simulink model "bh_explore_speed_control_and_manoeuvres"  (R2018a)
settings: Solver=ode45  StartTime=0.0  StopTime=15  FixedStep=0.001  RelTol=1e-5
undefined symbols (not defined in the file or in its folder): sigbuilder_block
libraries: simulink_extras x14, bh_cv_car_drc_library x1
settings Model: Creator=bhorton  LastModifiedBy=bhorton
settings SolverCC: ZeroCrossControl=EnableAll  ZeroCrossAlgorithm=Adaptive
settings DebuggingCC: SignalInfNanChecking=warning
settings ModelReferenceCC: ModelReferenceMinAlgLoopOccurrences=on

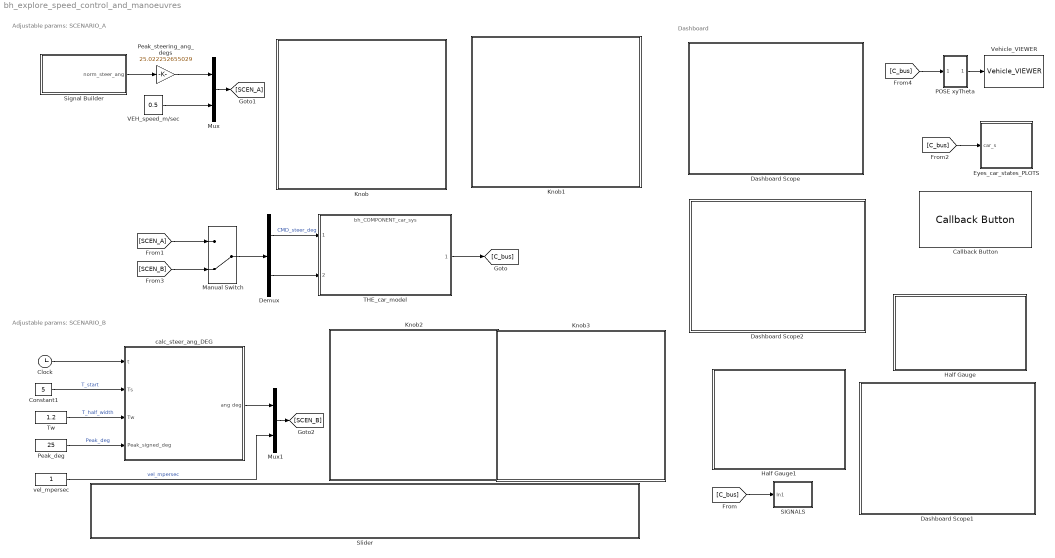
== system bh_explore_speed_control_and_manoeuvres ==
  note: Dashboard
  note: Adjustable params: SCENARIO_A
  note: Adjustable params: SCENARIO_B
  Callback Button : CallbackButton  WebBlockId=1673  PressFcn=""  ButtonText=OPEN State Plots
      settings: ClickFcn=|
      | open_system([bdroot,'/Eyes_car_states_PLOTS/car_states'])
      | open_system([bdroot,'/Eyes_car_states_PLOTS/Forces_BODY_frame'])
  Clock : Clock
  Constant1 : Constant  Value=5
  Dashboard Scope : Subsystem  DialogController=hmiCreateDDGDialog  IsWebBlock=on  mask(MWDashboardBlock){webBlockId=37415055-6488-43ff-9aef-d1c13ce01a1d, webBlockType=sdiscope, ShowInitialText=on, HMISrcModelName=bh_explore_speed_control_and_manoeuvres}
      mask prompts: webBlockId "WebBlock Id"; webBlockType "WebBlock Type"; HMISrcModelName "Source Model"
      mask help: SimulinkHMI:dialogs:HMIScopeDialogDesc
      mask Help: helpview([docroot '/mapfiles/simulink.map'], 'hmi_scope')
      mask Display:
      | if strcmp(get_param(bdroot(gcb),'BlockDiagramType'), 'library')
      |     image([(matlabroot) '/toolbox/simulink/hmi/icons/DashboardScope.png']);
      | end
  Dashboard Scope1 : Subsystem  DialogController=hmiCreateDDGDialog  IsWebBlock=on  mask(MWDashboardBlock){webBlockId=0f87227d-f9f9-4bc4-b6ae-007699aa5c2c, webBlockType=sdiscope, ShowInitialText=on, HMISrcModelName=bh_explore_speed_control_and_manoeuvres}
      mask prompts: webBlockId "WebBlock Id"; webBlockType "WebBlock Type"; HMISrcModelName "Source Model"
      mask help: SimulinkHMI:dialogs:HMIScopeDialogDesc
      mask Help: helpview([docroot '/mapfiles/simulink.map'], 'hmi_scope')
      mask Display:
      | if strcmp(get_param(bdroot(gcb),'BlockDiagramType'), 'library')
      |     image([(matlabroot) '/toolbox/simulink/hmi/icons/DashboardScope.png']);
      | end
  Dashboard Scope2 : Subsystem  DialogController=hmiCreateDDGDialog  IsWebBlock=on  mask(MWDashboardBlock){webBlockId=6b014668-cd52-46a0-a1ab-7f5af930874b, webBlockType=sdiscope, ShowInitialText=on, HMISrcModelName=bh_explore_speed_control_and_manoeuvres}
      mask prompts: webBlockId "WebBlock Id"; webBlockType "WebBlock Type"; HMISrcModelName "Source Model"
      mask help: SimulinkHMI:dialogs:HMIScopeDialogDesc
      mask Help: helpview([docroot '/mapfiles/simulink.map'], 'hmi_scope')
      mask Display:
      | if strcmp(get_param(bdroot(gcb),'BlockDiagramType'), 'library')
      |     image([(matlabroot) '/toolbox/simulink/hmi/icons/DashboardScope.png']);
      | end
  Demux : Demux  Outputs=2
  Eyes_car_states_PLOTS : Subsystem
  Half Gauge : Subsystem  DialogController=hmiCreateDDGDialog  IsWebBlock=on  mask(MWDashboardBlock){webBlockId=7d5ce28d-d875-432d-8f3a-719b52f1dd3d, webBlockType=semicirculargauge, ShowInLibBrowser=on, ShowInitialText=on, HMISrcModelName=bh_explore_speed_control_and_manoeuvres}
      mask prompts: webBlockId "WebBlock Id"; webBlockType "WebBlock Type"; HMISrcModelName "Source Model"
      mask help: SimulinkHMI:dialogs:SemicircularGaugeDialogDesc
      mask Help: helpview([docroot '/mapfiles/simulink.map'], 'hmi_half_gauge')
      mask Display:
      | if strcmp(get_param(bdroot(gcb),'BlockDiagramType'), 'library')
      |     image([(matlabroot) '/toolbox/simulink/hmi/icons/SemicircularGauge.png']);
      | end
  Half Gauge1 : Subsystem  DialogController=hmiCreateDDGDialog  IsWebBlock=on  mask(MWDashboardBlock){webBlockId=b5d4b91a-5326-4bfa-bfd5-f4d409ef95d8, webBlockType=semicirculargauge, ShowInLibBrowser=on, ShowInitialText=on, HMISrcModelName=bh_explore_speed_control_and_manoeuvres}
      mask prompts: webBlockId "WebBlock Id"; webBlockType "WebBlock Type"; HMISrcModelName "Source Model"
      mask help: SimulinkHMI:dialogs:SemicircularGaugeDialogDesc
      mask Help: helpview([docroot '/mapfiles/simulink.map'], 'hmi_half_gauge')
      mask Display:
      | if strcmp(get_param(bdroot(gcb),'BlockDiagramType'), 'library')
      |     image([(matlabroot) '/toolbox/simulink/hmi/icons/SemicircularGauge.png']);
      | end
  Knob : Subsystem  DialogController=hmiCreateDDGDialog  IsWebBlock=on  mask(MWDashboardBlock){webBlockId=3ae3ec89-5f06-4569-b08b-ae0e4db549b5, webBlockType=continuousknob, ShowInLibBrowser=on, ShowInitialText=on, HMISrcModelName=bh_explore_speed_control_and_manoeuvres}
      mask prompts: webBlockId "WebBlock Id"; webBlockType "WebBlock Type"; HMISrcModelName "Source Model"
      mask help: SimulinkHMI:dialogs:ContinuousKnobDialogDesc
      mask Help: helpview([docroot '/mapfiles/simulink.map'], 'hmi_knob')
      mask Display:
      | if strcmp(get_param(bdroot(gcb),'BlockDiagramType'), 'library')
      |     image([(matlabroot) '/toolbox/simulink/hmi/icons/ContinuousKnob.png']);
      | end
  Knob1 : Subsystem  DialogController=hmiCreateDDGDialog  IsWebBlock=on  mask(MWDashboardBlock){webBlockId=ad926c90-b8a8-45cf-ba7e-52fdfa91ce01, webBlockType=continuousknob, ShowInLibBrowser=on, ShowInitialText=on, HMISrcModelName=bh_explore_speed_control_and_manoeuvres}
      mask prompts: webBlockId "WebBlock Id"; webBlockType "WebBlock Type"; HMISrcModelName "Source Model"
      mask help: SimulinkHMI:dialogs:ContinuousKnobDialogDesc
      mask Help: helpview([docroot '/mapfiles/simulink.map'], 'hmi_knob')
      mask Display:
      | if strcmp(get_param(bdroot(gcb),'BlockDiagramType'), 'library')
      |     image([(matlabroot) '/toolbox/simulink/hmi/icons/ContinuousKnob.png']);
      | end
  Knob2 : Subsystem  DialogController=hmiCreateDDGDialog  IsWebBlock=on  mask(MWDashboardBlock){webBlockId=2668dcc9-a1cd-4bf1-9da4-0c933115db1b, webBlockType=continuousknob, ShowInLibBrowser=on, ShowInitialText=on, HMISrcModelName=bh_explore_speed_control_and_manoeuvres}
      mask prompts: webBlockId "WebBlock Id"; webBlockType "WebBlock Type"; HMISrcModelName "Source Model"
      mask help: SimulinkHMI:dialogs:ContinuousKnobDialogDesc
      mask Help: helpview([docroot '/mapfiles/simulink.map'], 'hmi_knob')
      mask Display:
      | if strcmp(get_param(bdroot(gcb),'BlockDiagramType'), 'library')
      |     image([(matlabroot) '/toolbox/simulink/hmi/icons/ContinuousKnob.png']);
      | end
  Knob3 : Subsystem  DialogController=hmiCreateDDGDialog  IsWebBlock=on  mask(MWDashboardBlock){webBlockId=14dcc02d-a3fe-4bd7-90d9-1a858d2b9cd1, webBlockType=continuousknob, ShowInLibBrowser=on, ShowInitialText=on, HMISrcModelName=bh_explore_speed_control_and_manoeuvres}
      mask prompts: webBlockId "WebBlock Id"; webBlockType "WebBlock Type"; HMISrcModelName "Source Model"
      mask help: SimulinkHMI:dialogs:ContinuousKnobDialogDesc
      mask Help: helpview([docroot '/mapfiles/simulink.map'], 'hmi_knob')
      mask Display:
      | if strcmp(get_param(bdroot(gcb),'BlockDiagramType'), 'library')
      |     image([(matlabroot) '/toolbox/simulink/hmi/icons/ContinuousKnob.png']);
      | end
  Manual Switch : ManualSwitch  CurrentSetting=0
  Mux : Mux  Inputs=2
  Mux1 : Mux  Inputs=2
  POSE xyTheta : Subsystem
  Peak_deg : Constant  Value=25
  Peak_steering_ang_degs : Gain  Gain=25.022252655029
  SIGNALS : Subsystem
  Signal Builder : Subsystem  Tag=STV Subsys  LoadFcn=sigbuilder_block('load');  StartFcn=sigbuilder_block('start');  StopFcn=sigbuilder_block('stop');  ClipboardFcn=sigbuilder_block('clipboard');  mask(Sigbuilder block){tuvar=[0:10]}
      mask help: Simulink:masks:SigbuilderBlock_MD
      mask init:
      | if ~strcmp(get_param(bdroot(gcbh),'SimulationStatus'),'stopped') tuvar = sigbuilder_block('maskInit'); end
      settings: CopyFcn=sigbuilder_block('copy');  DeleteFcn=sigbuilder_block('delete');  ModelCloseFcn=sigbuilder_block('modelClose');  PreSaveFcn=sigbuilder_block('preSave');  PauseFcn=sigbuilder_block('pause');  ContinueFcn=sigbuilder_block('continue');  NameChangeFcn=sigbuilder_block('namechange');  OpenFcn=sigbuilder_block('open',[6 24.75 1428 637.5 ]);  CloseFcn=sigbuilder_block('close');
      mask Display: plot(0, 0, 100, 100,[2, 2, 32, 32, 2], [68, 8, 8, 68, 68],[32, 2], [38, 38], [32, 19, 2],[53, 60, 44], [32, 17, 17, 2],[16, 16, 31, 31]);txt = getActiveGroup(gcbh);text(2, 100, txt,'verticalAlignment', 'top');
  Slider : Subsystem  DialogController=hmiCreateDDGDialog  IsWebBlock=on  mask(MWDashboardBlock){webBlockId=1f65ddbe-eef6-400e-a434-9b8f03db9885, webBlockType=slider, ShowInLibBrowser=on, ShowInitialText=on, HMISrcModelName=bh_explore_speed_control_and_manoeuvres}
      mask prompts: webBlockId "WebBlock Id"; webBlockType "WebBlock Type"; HMISrcModelName "Source Model"
      mask help: SimulinkHMI:dialogs:SliderDialogDesc
      mask Help: helpview([docroot '/mapfiles/simulink.map'], 'hmi_slider')
      mask Display:
      | if strcmp(get_param(bdroot(gcb),'BlockDiagramType'), 'library')
      |     image([(matlabroot) '/toolbox/simulink/hmi/icons/Slider.png']);
      | end
  THE_car_model : ModelReference  ModelNameDialog=bh_COMPONENT_car_sys  SimulationMode=Normal  ModelReferenceVersion=1.273
  Tw : Constant  Value=1.2
  VEH_speed_m/sec : Constant  Value=0.5
  Vehicle_VIEWER : bh_cv_car_drc_library/CAR_things/Vehicle_VIEWER  wp_mat=[-1, -1; 2,2]  veh_ID_num=1  veh_init_xytheta=[0,0,0]  Ts=0.1
  calc_steer_ang_DEG : Subsystem
      mask Display: image(imread('evassive_PIC_01.JPG'))
  vel_mpersec : Constant
  wires:
  [C_bus] -> Eyes_car_states_PLOTS/1(car_s)
  THE_car_model/1 -> [C_bus]
  [C_bus] -> POSE xyTheta/1(In1)
  POSE xyTheta/1(Out1) -> Vehicle_VIEWER/1
  Signal Builder/1(norm_steer_ang) -> Peak_steering_ang_degs/1
  Peak_steering_ang_degs/1 -> Mux/1
  [C_bus] -> SIGNALS/1(In1)
  VEH_speed_m/sec/1 -> Mux/2
  Manual Switch/1 -> Demux/1
  Demux/1 -> THE_car_model/1  "CMD_steer_deg"
  Demux/2 -> THE_car_model/2
  [SCEN_A] -> Manual Switch/1
  Mux/1 -> [SCEN_A]
  Peak_deg/1 -> calc_steer_ang_DEG/4(Peak_signed_deg)  "Peak_deg"
  Constant1/1 -> calc_steer_ang_DEG/2(Ts)  "T_start"
  Clock/1 -> calc_steer_ang_DEG/1(t)
  Mux1/1 -> [SCEN_B]
  calc_steer_ang_DEG/1(ang deg) -> Mux1/1
  vel_mpersec/1 -> Mux1/2  "vel_mpersec"
  Tw/1 -> calc_steer_ang_DEG/3(Tw)  "T_half_width"
  [SCEN_B] -> Manual Switch/2

== system bh_explore_speed_control_and_manoeuvres/Dashboard Scope ==

== system bh_explore_speed_control_and_manoeuvres/Dashboard Scope1 ==

== system bh_explore_speed_control_and_manoeuvres/Dashboard Scope2 ==

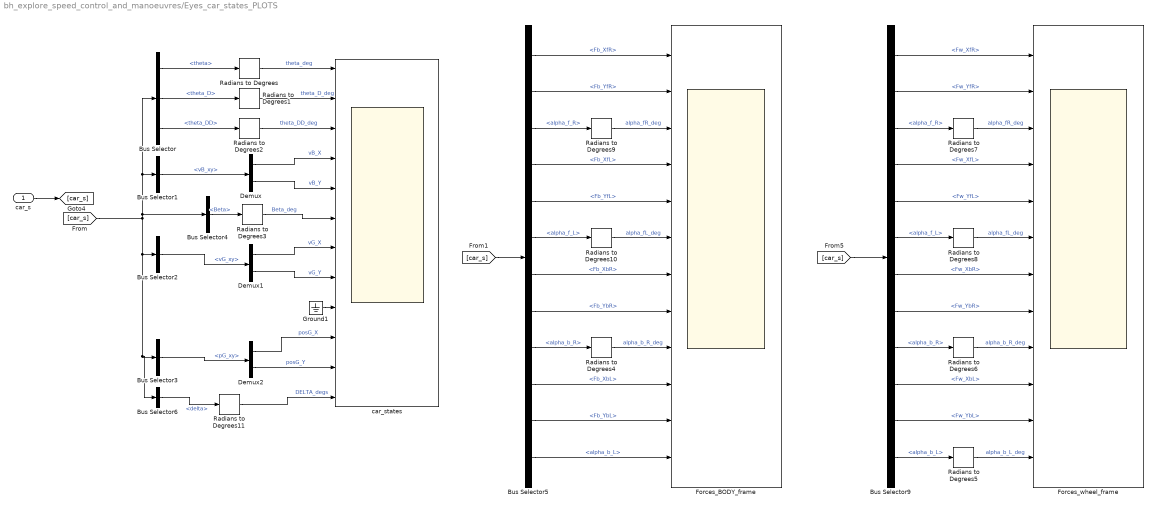
== system bh_explore_speed_control_and_manoeuvres/Eyes_car_states_PLOTS ==
  car_s : Inport
  Bus Selector : BusSelector  OutputSignals=states_B.theta,states_B.theta_D,states_B.theta_DD
  Bus Selector1 : BusSelector  OutputSignals=states_B.vB_xy
  Bus Selector2 : BusSelector  OutputSignals=states_G.vG_xy
  Bus Selector3 : BusSelector  OutputSignals=states_G.pG_xy
  Bus Selector4 : BusSelector  OutputSignals=states_B.Beta
  Bus Selector5 : BusSelector  OutputSignals=Force_BODY_frame.Fb_XfR,Force_BODY_frame.Fb_YfR,alpha.alpha_f_R,Force_BODY_frame.Fb_XfL,Force_BODY_frame.Fb_YfL,alpha.alpha_f_L,Force_BODY_frame.Fb_XbR,Force_BODY_frame.Fb_YbR,alpha.alpha_b_R,Force_BODY_frame.Fb_XbL,Force_BODY_frame.Fb_YbL,alpha.alpha_b_L
  Bus Selector6 : BusSelector  OutputSignals=wheel.delta
  Bus Selector9 : BusSelector  OutputSignals=Force_wheel_frame.Fw_XfR,Force_wheel_frame.Fw_YfR,alpha.alpha_f_R,Force_wheel_frame.Fw_XfL,Force_wheel_frame.Fw_YfL,alpha.alpha_f_L,Force_wheel_frame.Fw_XbR,Force_wheel_frame.Fw_YbR,alpha.alpha_b_R,Force_wheel_frame.Fw_XbL,Force_wheel_frame.Fw_YbL,alpha.alpha_b_L
  Demux : Demux  Outputs=2
  Demux1 : Demux  Outputs=2
  Demux2 : Demux  Outputs=2
  Forces_BODY_frame : Scope  NumInputPorts=12
  Forces_wheel_frame : Scope  NumInputPorts=12
  Ground1 : Ground
  Radians to Degrees{,1..11} (12 alike) : simulink_extras/Transformations/Radians to Degrees
  car_states : Scope  NumInputPorts=12
  wires:
  car_s/1 -> [car_s]
  [car_s] -> Bus Selector4/1, Bus Selector/1, Bus Selector1/1, Bus Selector6/1, Bus Selector3/1, Bus Selector2/1
  Bus Selector/1 -> Radians to Degrees/1  "<theta>"
  Bus Selector/2 -> Radians to Degrees1/1  "<theta_D>"
  Bus Selector/3 -> Radians to Degrees2/1  "<theta_DD>"
  Radians to Degrees/1 -> car_states/1  "theta_deg"
  Radians to Degrees1/1 -> car_states/2  "theta_D_deg"
  Radians to Degrees2/1 -> car_states/3  "theta_DD_deg"
  Bus Selector1/1 -> Demux/1  "<vB_xy>"
  Demux/1 -> car_states/4  "vB_X"
  Demux/2 -> car_states/5  "vB_Y"
  Radians to Degrees3/1 -> car_states/6  "Beta_deg"
  Bus Selector2/1 -> Demux1/1  "<vG_xy>"
  Demux1/1 -> car_states/7  "vG_X"
  Demux1/2 -> car_states/8  "vG_Y"
  Ground1/1 -> car_states/9
  Demux2/1 -> car_states/10  "posG_X"
  Demux2/2 -> car_states/11  "posG_Y"
  Bus Selector3/1 -> Demux2/1  "<pG_xy>"
  Radians to Degrees11/1 -> car_states/12  "DELTA_degs"
  Bus Selector4/1 -> Radians to Degrees3/1  "<Beta>"
  [car_s] -> Bus Selector9/1
  Bus Selector9/1 -> Forces_wheel_frame/1  "<Fw_XfR>"
  Bus Selector9/2 -> Forces_wheel_frame/2  "<Fw_YfR>"
  Bus Selector9/3 -> Radians to Degrees7/1  "<alpha_f_R>"
  Bus Selector9/4 -> Forces_wheel_frame/4  "<Fw_XfL>"
  Bus Selector9/5 -> Forces_wheel_frame/5  "<Fw_YfL>"
  Bus Selector9/6 -> Radians to Degrees8/1  "<alpha_f_L>"
  Bus Selector9/7 -> Forces_wheel_frame/7  "<Fw_XbR>"
  Bus Selector9/8 -> Forces_wheel_frame/8  "<Fw_YbR>"
  Bus Selector9/9 -> Radians to Degrees6/1  "<alpha_b_R>"
  Bus Selector9/10 -> Forces_wheel_frame/10  "<Fw_XbL>"
  Bus Selector9/11 -> Forces_wheel_frame/11  "<Fw_YbL>"
  Bus Selector9/12 -> Radians to Degrees5/1  "<alpha_b_L>"
  Radians to Degrees7/1 -> Forces_wheel_frame/3  "alpha_fR_deg"
  Radians to Degrees8/1 -> Forces_wheel_frame/6  "alpha_fL_deg"
  Radians to Degrees6/1 -> Forces_wheel_frame/9  "alpha_b_R_deg"
  Radians to Degrees5/1 -> Forces_wheel_frame/12  "alpha_b_L_deg"
  Radians to Degrees10/1 -> Forces_BODY_frame/6  "alpha_fL_deg"
  Radians to Degrees4/1 -> Forces_BODY_frame/9  "alpha_b_R_deg"
  Radians to Degrees9/1 -> Forces_BODY_frame/3  "alpha_fR_deg"
  Bus Selector5/9 -> Radians to Degrees4/1  "<alpha_b_R>"
  Bus Selector5/7 -> Forces_BODY_frame/7  "<Fb_XbR>"
  Bus Selector5/10 -> Forces_BODY_frame/10  "<Fb_XbL>"
  Bus Selector5/11 -> Forces_BODY_frame/11  "<Fb_YbL>"
  Bus Selector5/6 -> Radians to Degrees10/1  "<alpha_f_L>"
  Bus Selector5/5 -> Forces_BODY_frame/5  "<Fb_YfL>"
  Bus Selector5/4 -> Forces_BODY_frame/4  "<Fb_XfL>"
  Bus Selector5/8 -> Forces_BODY_frame/8  "<Fb_YbR>"
  Bus Selector5/2 -> Forces_BODY_frame/2  "<Fb_YfR>"
  [car_s] -> Bus Selector5/1
  Bus Selector5/3 -> Radians to Degrees9/1  "<alpha_f_R>"
  Bus Selector5/1 -> Forces_BODY_frame/1  "<Fb_XfR>"
  Bus Selector5/12 -> Forces_BODY_frame/12  "<alpha_b_L>"
  Bus Selector6/1 -> Radians to Degrees11/1  "<delta>"

== system bh_explore_speed_control_and_manoeuvres/Half Gauge ==

== system bh_explore_speed_control_and_manoeuvres/Half Gauge1 ==

== system bh_explore_speed_control_and_manoeuvres/Knob ==

== system bh_explore_speed_control_and_manoeuvres/Knob1 ==

== system bh_explore_speed_control_and_manoeuvres/Knob2 ==

== system bh_explore_speed_control_and_manoeuvres/Knob3 ==

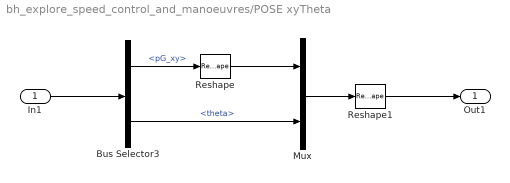
== system bh_explore_speed_control_and_manoeuvres/POSE xyTheta ==
  In1 : Inport
  Bus Selector3 : BusSelector  OutputSignals=states_G.pG_xy,states_B.theta
  Mux : Mux  Inputs=2
  Reshape : Reshape  OutputDimensionality=Column vector (2-D)
  Reshape1 : Reshape  OutputDimensionality=Column vector (2-D)
  Out1 : Outport
  wires:
  In1/1 -> Bus Selector3/1
  Bus Selector3/1 -> Reshape/1  "<pG_xy>"
  Reshape/1 -> Mux/1
  Bus Selector3/2 -> Mux/2  "<theta>"
  Mux/1 -> Reshape1/1
  Reshape1/1 -> Out1/1

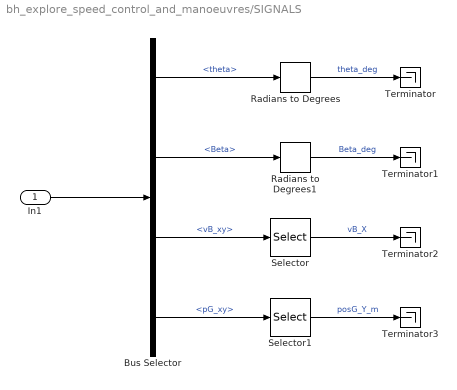
== system bh_explore_speed_control_and_manoeuvres/SIGNALS ==
  In1 : Inport
  Bus Selector : BusSelector  OutputSignals=states_B.theta,states_B.Beta,states_B.vB_xy,states_G.pG_xy
  Radians to Degrees : simulink_extras/Transformations/Radians to Degrees
  Radians to Degrees1 : simulink_extras/Transformations/Radians to Degrees
  Selector : Selector  InputPortWidth=2  IndexOptions=Index vector (dialog)  Indices=1  OutputSizes=1
  Selector1 : Selector  InputPortWidth=2  IndexOptions=Index vector (dialog)  Indices=2  OutputSizes=1
  Terminator{,1..3} (4 alike) : Terminator
  wires:
  In1/1 -> Bus Selector/1
  Bus Selector/1 -> Radians to Degrees/1  "<theta>"
  Bus Selector/2 -> Radians to Degrees1/1  "<Beta>"
  Bus Selector/3 -> Selector/1  "<vB_xy>"
  Selector/1 -> Terminator2/1  "vB_X"
  Bus Selector/4 -> Selector1/1  "<pG_xy>"
  Selector1/1 -> Terminator3/1  "posG_Y_m"
  Radians to Degrees/1 -> Terminator/1  "theta_deg"
  Radians to Degrees1/1 -> Terminator1/1  "Beta_deg"

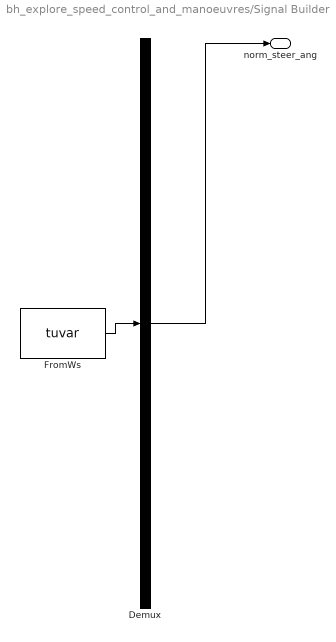
== system bh_explore_speed_control_and_manoeuvres/Signal Builder ==
  Demux : Demux  Tag=STV Demux  Outputs=1
  FromWs : FromWorkspace  Tag=STV FromWs  VariableName=tuvar  SampleTime=0
      SigBuilderData=|
      | common.afterFinalStr = 'Extrapolate'
      | common.sampleTime = 0
      | dataSet(1).timeRange = [0 60]
      | dataSet(1).name = 'turn_then_center'
      | dataSet(2).timeRange = [0 60]
      | dataSet(2).name = 'TC_TC_01'
      | dataSet(3).timeRange = [0 60]
      | dataSet(3).name = 'TC_TC_02'
      | dataSet(4).timeRange = [0 60]
      | dataSet(4).name = 'TC_A'
      | dataSet(5).timeRange = [0 60]
      | dataSet(5).name = 'Step'
      | dataSet(6).timeRange = [0 60]
      | dataSet(6).name = 'Straight'
      | dataSet(7).timeRange = [0 60]
      | dataSet(7).name = 'TC_TC_3'
      | dataSet(8).timeRange = [0 60]
      | dataSet(8).name = 'Straight_FULL_LOCK'
      | sbobj.Groups(1).Name = 'turn_then_center'
      | sbobj.Groups(1).Signals.Name = 'norm_steer_ang'
      | sbobj.Groups(1).Signals.XData = [0 10.05 10.05 14 14 60]
      | sbobj.Groups(1).Signals.YData = [0 0 1 1 0 0]
      | sbobj.Groups(1).TimeRange = [0 60]
      | sbobj.Groups(2).Name = 'TC_TC_01'
      | sbobj.Groups(2).Signals.Name = 'norm_steer_ang'
      | sbobj.Groups(2).Signals.XData = [0 20.1 25 30 35 40 60]
      | sbobj.Groups(2).Signals.YData = [0 0 1 0 -1 0 0]
      | sbobj.Groups(2).TimeRange = [0 60]
      | sbobj.Groups(3).Name = 'TC_TC_02'
      | sbobj.Groups(3).Signals.Name = 'norm_steer_ang'
      | sbobj.Groups(3).Signals.XData = [0 20.1 21 22 23 24 60]
      | sbobj.Groups(3).Signals.YData = [0 0 1 0 -1 0 0]
      | sbobj.Groups(3).TimeRange = [0 60]
      | sbobj.Groups(4).Name = 'TC_A'
      | sbobj.Groups(4).Signals.Name = 'norm_steer_ang'
      | sbobj.Groups(4).Signals.XData = [0 20.1 30 40 60]
      | sbobj.Groups(4).Signals.YData = [0 0 1 0 0]
      | sbobj.Groups(4).TimeRange = [0 60]
      | sbobj.Groups(5).Name = 'Step'
      | sbobj.Groups(5).Signals.Name = 'norm_steer_ang'
      | sbobj.Groups(5).Signals.XData = [0 20 20.1 60]
      | sbobj.Groups(5).Signals.YData = [0 0 1 1]
      | sbobj.Groups(5).TimeRange = [0 60]
      | sbobj.Groups(6).Name = 'Straight'
      | sbobj.Groups(6).Signals.Name = 'norm_steer_ang'
      | sbobj.Groups(6).Signals.XData = [0 60]
      | sbobj.Groups(6).Signals.YData = [0 0]
      | sbobj.Groups(6).TimeRange = [0 60]
      | sbobj.Groups(7).Name = 'TC_TC_3'
      | sbobj.Groups(7).Signals.Name = 'norm_steer_ang'
      | sbobj.Groups(7).Signals.XData = [0 10 11 12 13 14 60]
      | sbobj.Groups(7).Signals.YData = [0 0 1 0 -1 0 0]
      | sbobj.Groups(7).TimeRange = [0 60]
      | sbobj.Groups(8).Name = 'Straight_FULL_LOCK'
      | sbobj.Groups(8).Signals.Name = 'norm_steer_ang'
      | sbobj.Groups(8).Signals.XData = [0 10 10 60]
      | sbobj.Groups(8).Signals.YData = [0 0 1 1]
      | sbobj.Groups(8).TimeRange = [0 60]
  norm_steer_ang : Outport  Tag=STV Outport
  wires:
  Demux/1 -> norm_steer_ang/1
  FromWs/1 -> Demux/1

== system bh_explore_speed_control_and_manoeuvres/Slider ==

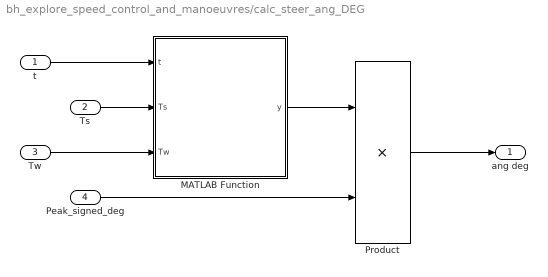
== system bh_explore_speed_control_and_manoeuvres/calc_steer_ang_DEG ==
  t : Inport
  Ts : Inport  Port=2
  Tw : Inport  Port=3
  Peak_signed_deg : Inport  Port=4
  MATLAB Function : MATLAB Function  TreatAsAtomicUnit=on
  Product : Product
  ang deg : Outport
  wires:
  t/1 -> MATLAB Function/1(t)
  Ts/1 -> MATLAB Function/2(Ts)
  Tw/1 -> MATLAB Function/3(Tw)
  MATLAB Function/1(y) -> Product/1
  Peak_signed_deg/1 -> Product/2
  Product/1 -> ang deg/1

== matlab function bh_explore_speed_control_and_manoeuvres/calc_steer_ang_DEG/MATLAB Function ==
  data: t input; y output; Ts input; Tw input
function y = fcn(t,Ts,Tw)

y = 0;

% first look for the out of bounds cases
if(  t <= Ts )
    return;
end

if( t >= (Ts + 2*Tw) )
    return;
end

%OK: if we're here then do your thing
m_climbing = 1/(Tw/2);
m_falling  = -1 * m_climbing;

if(  (t > Ts) && (t <= (Ts + Tw/2))  )
    % first CLIMBING zone
    t_star = t - Ts;
         y = t_star * m_climbing;
elseif(  (t > (Ts + Tw/2)) && (t <= (Ts + 3*Tw/2))   )
    % the FALLING zone
    t_star = t - (Ts + Tw/2);
         y = t_star * m_falling +  1;
else
    % the 2nd CLIMBING zone
    t_star = t - (Ts + 3*Tw/2);
         y = t_star * m_climbing -  1;
end
